simulink library "ddm"  (R2021b)
settings: Solver=VariableStepAuto  StartTime=0.0  StopTime=10.0  RelTol=1e-3
undefined symbols (not defined in the file or in its folder): ADDM_FrTMTqDev_X_Nm, ADDM_RrTMTqDev_X_Nm, ENUM_ADASACCSTA_ERROR, ENUM_ADASACCSTA_OFF, ENUM_ADASACCSTA_STANDBY, ENUM_ALLOWMOV_ALLOWREADY, ENUM_APS, ENUM_BRKSTA_ERROR, ENUM_BRKSTA_OFF, ENUM_BRKSTA_ON, ENUM_BRKSW_INVALID, ENUM_BRKSW_OFF, ENUM_BRKSW_ON, ENUM_CHGPREACTERRSTA_OBCPRE, ENUM_DCDCFAULTSTA_ANYFAULTLV1, ENUM_DCDCFAULTSTA_ANYFAULTLV2, ENUM_DRIVETRAIN_AWD, ENUM_DRIVETRAIN_FWD, ENUM_DRIVETRAIN_RWD, ENUM_EDUDRTSTA_NORMAL, ENUM_EPBSTA_APPLIED, ENUM_EPBSTA_RELEASED, ENUM_GEARACTUALPOSN_INVALID, ENUM_GEARACTUALPOSN_P, ENUM_HVBATTREADYPRE_READY, ENUM_MCUWARN_LV0, ENUM_MCUWARN_LV1, ENUM_MCUWARN_LV2, ENUM_MCUWARN_LV3, ENUM_MCUWARN_NOERROR, ENUM_OBCFAULTSTA_ANYFAULT, ENUM_PAS_R2F2, ENUM_PDFAULT_BATTPDFAIL, ENUM_PDFAULT_DCDCDISABLE, ENUM_PDFAULT_MCUDISABLE, ENUM_PDFAULT_MCUDISCHRG, ENUM_POWERSTA_OFF, ENUM_POWERSTA_ON, ENUM_POWERSTA_READY, ENUM_POWERSTA_STANDBY, ENUM_PRESSINDI_LOW, ENUM_PUFAULT_BATTUPFAIL, ENUM_PUFAULT_DCDCENABLEFAIL, ENUM_PUFAULT_PRECHRGCHKFAIL, ENUM_PUFAULT_SAFETYCHKFAIL, ENUM_PUSTATE_COMPLETED, ENUM_PWRSTASW_OFF, ENUM_PWRSTASW_OFFA, ENUM_PWRSTASW_OFFCHVCHRG, ENUM_PWRSTASW_OFFCLVCHRG, ENUM_PWRSTASW_ON, ENUM_PWRSTASW_ONHVCHRG, ENUM_PWRSTASW_READY, ENUM_PWRSTASW_STANDBY, ENUM_SHIFTCOMMAND_P, ENUM_SHIFTERERRSTA_PBUTTONFAILURE, ENUM_VEHMALFUNLV_2ND, ENUM_VEHMALFUNLV_3RD, ENUM_VEHMALFUNLV_4TH, ENUM_VEHMALFUNLV_NORMAL ... (+459)
libraries: hcu_lib x515, simulink x3
(part 9 of 25)

== system ddm/DDM/DDM/PMM/SW failure ==
  task_time_s : Inport
  VPMM_PwrStaSW_enum : Inport  Port=2
  VPMM_PowerSta_enum : Inport  Port=3
  DTC_clear_request : Inport  Port=4
  VINP_DrStSW : Inport  Port=5
  VINP_FLAJARSW : Inport  Port=6
  VINP_FRAJARSW : Inport  Port=7
  VINP_RLAJARSW : Inport  Port=8
  VINP_RRAJARSW : Inport  Port=9
  VINP_HoodSW : Inport  Port=10
  VINP_TailgaSW : Inport  Port=11
  Driver seat switch failure : Subsystem
  FL Door switch failure : Subsystem
  FR Door switch failure : Subsystem
  Hood switch failure : Subsystem
  RL Door switch failure : Subsystem
  RR Door switch failure : Subsystem
  Tailgate switch failure : Subsystem
  VDDM_DrStSWDTC_raw32 : Outport
  VDDM_FLDoorSWDTC_raw32 : Outport  Port=2
  VDDM_RLDoorSWDTC_raw32 : Outport  Port=3
  VDDM_FRDoorSWDTC_raw32 : Outport  Port=4
  VDDM_RRDoorSWDTC_raw32 : Outport  Port=5
  VDDM_HoodSWDTC_raw32 : Outport  Port=6
  VDDM_TailgaSWDTC_raw32 : Outport  Port=7
  VDDM_VCUFLDoorSta_flg : Outport  Port=8
  VDDM_VCUFRDoorSta_flg : Outport  Port=9
  VDDM_VCURLDoorSta_flg : Outport  Port=10
  VDDM_VCURRDoorSta_flg : Outport  Port=11
  VDDM_VCUHoodSWSta_flg : Outport  Port=12
  VDDM_VCUTailgateSWSta_flg : Outport  Port=13
  VDDM_DrStSWCFS_flg : Outport  Port=14
  VDDM_FLDoorSWCFS_flg : Outport  Port=15
  VDDM_RLDoorSWCFS_flg : Outport  Port=16
  VDDM_FRDoorSWCFS_flg : Outport  Port=17
  VDDM_RRDoorSWCFS_flg : Outport  Port=18
  VDDM_HoodSWCFS_flg : Outport  Port=19
  VDDM_TailgaSWCFS_flg : Outport  Port=20
  wires:
  Tailgate switch failure/2(VDDM_VCUTailgateSWSta_flg) -> VDDM_VCUTailgateSWSta_flg/1
  Tailgate switch failure/1(VDDM_TailgaSWDTC_raw32) -> VDDM_TailgaSWDTC_raw32/1
  [VINP_TailgaSW] -> Tailgate switch failure/4(VINP_TailgaSW)
  [DTC_clear_request] -> Tailgate switch failure/5(DTC_clear_request)
  [VPMM_PwrStaSW_enum] -> Tailgate switch failure/3(VPMM_PwrStaSW_enum)
  [VPMM_PowerSta_enum] -> Tailgate switch failure/2(VPMM_PowerSta_enum)
  [task_time_s] -> Tailgate switch failure/1(task_time_s)
  Hood switch failure/2(VDDM_VCUHoodSWSta_flg) -> VDDM_VCUHoodSWSta_flg/1
  Hood switch failure/1(VDDM_HoodSWDTC_raw32) -> VDDM_HoodSWDTC_raw32/1
  [DTC_clear_request] -> Hood switch failure/5(DTC_clear_request)
  [VINP_HoodSW] -> Hood switch failure/4(VINP_HoodSW)
  VINP_TailgaSW/1 -> [VINP_TailgaSW]
  VINP_HoodSW/1 -> [VINP_HoodSW]
  [VPMM_PwrStaSW_enum] -> Hood switch failure/3(VPMM_PwrStaSW_enum)
  [VPMM_PowerSta_enum] -> Hood switch failure/2(VPMM_PowerSta_enum)
  [task_time_s] -> Hood switch failure/1(task_time_s)
  RR Door switch failure/2(VDDM_VCURRDoorSta_flg) -> VDDM_VCURRDoorSta_flg/1
  RR Door switch failure/1(VDDM_RRDoorSWDTC_raw32) -> VDDM_RRDoorSWDTC_raw32/1
  [DTC_clear_request] -> RR Door switch failure/5(DTC_clear_request)
  [VINP_RRAJARSW] -> RR Door switch failure/4(VINP_RRAJARSW)
  [VPMM_PwrStaSW_enum] -> RR Door switch failure/3(VPMM_PwrStaSW_enum)
  [VPMM_PowerSta_enum] -> RR Door switch failure/2(VPMM_PowerSta_enum)
  [task_time_s] -> RR Door switch failure/1(task_time_s)
  RL Door switch failure/2(VDDM_VCURLDoorSta_flg) -> VDDM_VCURLDoorSta_flg/1
  RL Door switch failure/1(VDDM_RLDoorSWDTC_raw32) -> VDDM_RLDoorSWDTC_raw32/1
  [DTC_clear_request] -> RL Door switch failure/5(DTC_clear_request)
  [VINP_RLAJARSW] -> RL Door switch failure/4(VINP_RLAJARSW)
  [task_time_s] -> RL Door switch failure/1(task_time_s)
  [VPMM_PowerSta_enum] -> RL Door switch failure/2(VPMM_PowerSta_enum)
  [VPMM_PwrStaSW_enum] -> RL Door switch failure/3(VPMM_PwrStaSW_enum)
  FR Door switch failure/2(VDDM_VCUFRDoorSta_flg) -> VDDM_VCUFRDoorSta_flg/1
  FR Door switch failure/1(VDDM_FRDoorSWDTC_raw32) -> VDDM_FRDoorSWDTC_raw32/1
  [DTC_clear_request] -> FR Door switch failure/5(DTC_clear_request)
  [VINP_FRAJARSW] -> FR Door switch failure/4(VINP_FRAJARSW)
  [VPMM_PwrStaSW_enum] -> FR Door switch failure/3(VPMM_PwrStaSW_enum)
  [VPMM_PowerSta_enum] -> FR Door switch failure/2(VPMM_PowerSta_enum)
  [task_time_s] -> FR Door switch failure/1(task_time_s)
  FL Door switch failure/2(VDDM_VCUFLDoorSta_flg) -> VDDM_VCUFLDoorSta_flg/1
  FL Door switch failure/1(VDDM_FLDoorSWDTC_raw32) -> VDDM_FLDoorSWDTC_raw32/1
  [DTC_clear_request] -> FL Door switch failure/5(DTC_clear_request)
  [VINP_FLAJARSW] -> FL Door switch failure/4(VINP_FLAJARSW)
  [VPMM_PwrStaSW_enum] -> FL Door switch failure/3(VPMM_PwrStaSW_enum)
  [VPMM_PowerSta_enum] -> FL Door switch failure/2(VPMM_PowerSta_enum)
  [task_time_s] -> FL Door switch failure/1(task_time_s)
  VINP_RRAJARSW/1 -> [VINP_RRAJARSW]
  VINP_RLAJARSW/1 -> [VINP_RLAJARSW]
  VINP_FRAJARSW/1 -> [VINP_FRAJARSW]
  VINP_FLAJARSW/1 -> [VINP_FLAJARSW]
  Driver seat switch failure/2(VDDM_DrStSWCFS_flg) -> VDDM_DrStSWCFS_flg/1
  DTC_clear_request/1 -> [DTC_clear_request]
  VPMM_PowerSta_enum/1 -> [VPMM_PowerSta_enum]
  VPMM_PwrStaSW_enum/1 -> [VPMM_PwrStaSW_enum]
  task_time_s/1 -> [task_time_s]
  VINP_DrStSW/1 -> [VINP_DrStSW]
  [task_time_s] -> Driver seat switch failure/1(task_time_s)
  [VINP_DrStSW] -> Driver seat switch failure/4(VINP_DrStSW)
  [DTC_clear_request] -> Driver seat switch failure/5(DTC_clear_request)
  [VPMM_PwrStaSW_enum] -> Driver seat switch failure/3(VPMM_PwrStaSW_enum)
  [VPMM_PowerSta_enum] -> Driver seat switch failure/2(VPMM_PowerSta_enum)
  Driver seat switch failure/1(VDDM_DrStSWDTC_raw32) -> VDDM_DrStSWDTC_raw32/1
  FL Door switch failure/3(VDDM_FLDoorSWCFS_flg) -> VDDM_FLDoorSWCFS_flg/1
  RL Door switch failure/3(VDDM_RLDoorSWCFS_flg) -> VDDM_RLDoorSWCFS_flg/1
  FR Door switch failure/3(VDDM_FRDoorSWCFS_flg) -> VDDM_FRDoorSWCFS_flg/1
  RR Door switch failure/3(VDDM_RRDoorSWCFS_flg) -> VDDM_RRDoorSWCFS_flg/1
  Hood switch failure/3(VDDM_HoodSWCFS_flg) -> VDDM_HoodSWCFS_flg/1
  Tailgate switch failure/3(VDDM_TailgaSWCFS_flg) -> VDDM_TailgaSWCFS_flg/1

== system ddm/DDM/DDM/PMM/System conditions of ON to READY not satisfied ==
  note: Release Condition After Decision
  note: Test Detection Criteria
  note: Diagnostics and Fault Handling
  note: Test Pass Criteria
  task_time_s : Inport
  VPMM_PowerSta_enum : Inport  Port=2
  VPMM_PwrStaSW_enum : Inport  Port=3
  DTC_clear_request : Inport  Port=4
  VPMM_MCUReady_flg : Inport  Port=5
  VINP_AllowMovThd_OTA_enum : Inport  Port=6
  VDDM_KeyAuthCFS_flg : Inport  Port=7
  VDDM_FLDoorSWCFS_flg : Inport  Port=8
  VDDM_RLDoorSWCFS_flg : Inport  Port=9
  VDDM_FRDoorSWCFS_flg : Inport  Port=10
  VDDM_RRDoorSWCFS_flg : Inport  Port=11
  VDDM_HoodSWCFS_flg : Inport  Port=12
  VDDM_TailgaSWCFS_flg : Inport  Port=13
  Constant{1..2,9,12,22} (5 alike) : Constant  Value=FALSE
  Constant10 : Constant  Value=ENUM_POWERSTA_STANDBY
  Constant13 : Constant  Value=KDDM_ONtoRdyPassTO_s
  Constant14 : Constant  Value=KDDM_ONtoRdyPassTO_s
  Constant17 : Constant  Value=KDDM_ONtoRdyDetTO_s
  Constant18 : Constant  Value=KDDM_ONtoRdyDTC_cnt
  Constant28 : Constant  Value=ENUM_PWRSTASW_ON
  Constant29 : Constant  Value=ENUM_PWRSTASW_ON
  Constant3 : Constant  Value=TRUE
  Constant30 : Constant  Value=KDDM_ONtoRdyDiagnosisOffSW_flg
  Constant31 : Constant  Value=ENUM_POWERSTA_OFF
  Constant32 : Constant  Value=ENUM_ALLOWMOV_ALLOWREADY
  Constant34 : Constant  Value=ZERO_INT
  Constant35 : Constant  Value=KDDM_ONtoRdyDTC_cnt
  Constant4 : Constant  Value=TRUE
  Constant5 : Constant  Value=ENUM_ALLOWMOV_ALLOWREADY
  DTC_Couter1 : hcu_lib/Basic_Blocks/DTC_Couter
  DTC_Info : hcu_lib/Basic_Blocks/DTC_Info
  Equal1 : RelationalOperator  Operator=~=  OutDataTypeStr=boolean  RndMeth=Simplest
  Equal{8,10,12,14} (4 alike) : RelationalOperator  Operator===  OutDataTypeStr=boolean  RndMeth=Simplest
  Equal11 : RelationalOperator  Operator=~=  OutDataTypeStr=boolean  RndMeth=Simplest
  Equal13 : RelationalOperator  OutDataTypeStr=boolean  RndMeth=Simplest
  Logical Operator1 : Logic  Operator=NOT  AllPortsSameDT=off  OutDataTypeStr=boolean
  Logical Operator14 : Logic  Operator=NOT  AllPortsSameDT=off  OutDataTypeStr=boolean
  Logical Operator16 : Logic  Operator=OR  Inputs=4  AllPortsSameDT=off  OutDataTypeStr=boolean
  Logical Operator17 : Logic  AllPortsSameDT=off  OutDataTypeStr=boolean
  Logical Operator2 : Logic  Operator=OR  Inputs=9  AllPortsSameDT=off  OutDataTypeStr=boolean
  Logical Operator20 : Logic  Operator=OR  Inputs=9  AllPortsSameDT=off  OutDataTypeStr=boolean
  Logical Operator21 : Logic  Operator=NOT  AllPortsSameDT=off  OutDataTypeStr=boolean
  Relational Operator1 : RelationalOperator  Operator=>  OutDataTypeStr=boolean  RndMeth=Simplest
  Switch{1..4,9} (5 alike) : Switch  Criteria=u2 ~= 0
  Terminator : Terminator
  Test Detection Criteria1 : hcu_lib/Basic_Blocks/Test Detection Criteria
  Timer2 : hcu_lib/Basic_Blocks/Timer
  Unit Delay1 : UnitDelay  SampleTime=-1  HasFrameUpgradeWarning=on
  VDDM_ONtoRdyDTC_raw32 : Outport
  VDDM_ONtoRdyCFS_flg : Outport  Port=2
  VDDM_EDriveSysErrONtoRdy_flg : Outport  Port=3
  VDDM_SysAllowReadySta_flg : Outport  Port=4
  wires:
  [VDDM_RRDoorSWCFS_flg] -> Logical Operator2/7
  Logical Operator2/1 -> Switch3/1
  [VDDM_FRDoorSWCFS_flg] -> Logical Operator2/6
  [VDDM_RLDoorSWCFS_flg] -> Logical Operator2/5
  [VDDM_FLDoorSWCFS_flg] -> Logical Operator2/4
  [VPMM_MCUReady_flg] -> Logical Operator1/1
  [VDDM_TailgaSWCFS_flg] -> Logical Operator2/9
  [VDDM_HoodSWCFS_flg] -> Logical Operator2/8
  [VDDM_KeyAuthCFS_flg] -> Logical Operator2/3
  Equal1/1 -> Logical Operator2/2
  Constant5/1 -> Equal1/2
  [VINP_AllowMovThd_OTA_enum] -> Equal1/1
  Logical Operator1/1 -> Logical Operator2/1
  [VDDM_TailgaSWCFS_flg] -> Logical Operator20/9
  [VDDM_HoodSWCFS_flg] -> Logical Operator20/8
  [VDDM_RRDoorSWCFS_flg] -> Logical Operator20/7
  [VDDM_FRDoorSWCFS_flg] -> Logical Operator20/6
  [VDDM_RLDoorSWCFS_flg] -> Logical Operator20/5
  [VDDM_FLDoorSWCFS_flg] -> Logical Operator20/4
  VDDM_TailgaSWCFS_flg/1 -> [VDDM_TailgaSWCFS_flg]
  VDDM_HoodSWCFS_flg/1 -> [VDDM_HoodSWCFS_flg]
  VDDM_RRDoorSWCFS_flg/1 -> [VDDM_RRDoorSWCFS_flg]
  VDDM_FRDoorSWCFS_flg/1 -> [VDDM_FRDoorSWCFS_flg]
  VDDM_RLDoorSWCFS_flg/1 -> [VDDM_RLDoorSWCFS_flg]
  VDDM_FLDoorSWCFS_flg/1 -> [VDDM_FLDoorSWCFS_flg]
  Switch4/1 -> VDDM_SysAllowReadySta_flg/1  "VDDM_SysAllowReadySta_flg"
  Constant1/1 -> Switch4/3
  Constant4/1 -> Switch4/1
  [VDDM_ONtoRdyCFS_flg] -> Switch4/2
  Switch2/1 -> VDDM_EDriveSysErrONtoRdy_flg/1  "VDDM_EDriveSysErrONtoRdy_flg"
  Constant3/1 -> Switch2/1
  Constant2/1 -> Switch2/3
  [VDDM_ONtoRdyCFS_flg] -> Switch2/2
  [VDDM_ONtoRdyCFS_flg] -> VDDM_ONtoRdyCFS_flg/1
  [VPMM_PwrStaSW_enum] -> Equal12/1
  Constant29/1 -> Equal12/2
  Constant9/1 -> Switch3/3
  Equal12/1 -> Switch3/2
  Constant32/1 -> Equal11/2
  [VDDM_KeyAuthCFS_flg] -> Logical Operator20/3
  Equal11/1 -> Logical Operator20/2
  Logical Operator14/1 -> Logical Operator20/1
  [VPMM_MCUReady_flg] -> Logical Operator14/1
  [VINP_AllowMovThd_OTA_enum] -> Equal11/1
  Logical Operator16/1 -> [VDDM_ONtoRdyCFSRls_flg]  "VDDM_ONtoRdyCFSRls_flg"
  [VDDM_ONtoRdyCFSRls_flg] -> DTC_Couter1/2
  [VDDM_ONtoRdyDet_flg] -> DTC_Couter1/1
  DTC_Couter1/1 -> [VDDM_ONtoRdyCFS_flg]  "VDDM_ONtoRdyCFS_flg"
  Constant14/1 -> Equal13/2
  [VDDM_ONtoRdyCFSRls_flg] -> Switch9/2
  Unit Delay1/1 -> Equal14/1
  Relational Operator1/1 -> Terminator/1  "VDDM_ONtoRdyDFS_flg"
  Constant34/1 -> Relational Operator1/2
  [VPMM_PowerSta_enum] -> Unit Delay1/1
  Equal14/1 -> Logical Operator17/1
  Switch3/1 -> Logical Operator21/1, Timer2/2
  Constant30/1 -> Logical Operator16/4
  Switch9/1 -> Test Detection Criteria1/1
  [task_time_s] -> Test Detection Criteria1/2
  [task_time_s] -> Timer2/3
  Switch1/1 -> Switch9/3
  Logical Operator21/1 -> Timer2/1
  Logical Operator17/1 -> Logical Operator16/1
  Constant12/1 -> Switch1/3
  Equal10/1 -> Logical Operator17/2
  Constant31/1 -> Equal14/2
  [DTC_clear_request] -> Logical Operator16/2
  DTC_Couter1/2 -> Relational Operator1/1  "VDDM_ONtoRdyDTC_cnt"
  Logical Operator20/1 -> Switch1/1
  [VPMM_PowerSta_enum] -> Equal10/1
  Constant22/1 -> Switch9/1
  Timer2/1 -> Equal13/1
  Constant10/1 -> Equal10/2
  Test Detection Criteria1/1 -> [VDDM_ONtoRdyDet_flg]  "VDDM_ONtoRdyDet_flg"
  Equal8/1 -> Switch1/2
  Constant13/1 -> Timer2/4
  Constant18/1 -> Test Detection Criteria1/3
  Constant35/1 -> DTC_Couter1/3
  [VPMM_PwrStaSW_enum] -> Equal8/1
  Equal13/1 -> [VDDM_ONtoRdyPass_flg]  "VDDM_ONtoRdyPass_flg"
  Constant28/1 -> Equal8/2
  Constant17/1 -> Test Detection Criteria1/4
  [VDDM_ONtoRdyPass_flg] -> Logical Operator16/3
  DTC_clear_request/1 -> [DTC_clear_request]
  task_time_s/1 -> [task_time_s]
  VPMM_PwrStaSW_enum/1 -> [VPMM_PwrStaSW_enum]
  VPMM_PowerSta_enum/1 -> [VPMM_PowerSta_enum]
  VPMM_MCUReady_flg/1 -> [VPMM_MCUReady_flg]
  VINP_AllowMovThd_OTA_enum/1 -> [VINP_AllowMovThd_OTA_enum]
  DTC_Info/1 -> VDDM_ONtoRdyDTC_raw32/1  "VDDM_ONtoRdyDTC_raw32"
  [VDDM_ONtoRdyPass_flg] -> DTC_Info/2
  [VDDM_ONtoRdyCFS_flg] -> DTC_Info/3
  VDDM_KeyAuthCFS_flg/1 -> [VDDM_KeyAuthCFS_flg]
  [VDDM_ONtoRdyDet_flg] -> DTC_Info/1
  [DTC_clear_request] -> DTC_Info/4

== system ddm/DDM/DDM/PMM/power up and power down ==
  note: Power up fail check
  note: Power down fail check
  note: OBC ready for precharge fail check
  task_time_s : Inport
  VPMM_PwrStaSW_enum : Inport  Port=2
  VPMM_PowerSta_enum : Inport  Port=3
  VPMM_PowerUpFault_enum : Inport  Port=4
  VPMM_PowerDownFault_enum : Inport  Port=5
  DTC_clear_request : Inport  Port=6
  VINP_HVBattReady4Pre_enum : Inport  Port=7
  VPMM_MCUReady4Pre_flg : Inport  Port=8
  VINP_DCDCReady4Pre_flg : Inport  Port=9
  VINP_HVBContactorSta_flg : Inport  Port=10
  VINP_BMSREADY_flg : Inport  Port=11
  VINP_DCDCEnabled_flg : Inport  Port=12
  VPMM_SafetyChkHLv_flg : Inport  Port=13
  VPMM_SafetyChkMLv_flg : Inport  Port=14
  VPMM_HVChrgPreActionErrSta_enum : Inport  Port=15
  VPMM_PowerUpState_enum : Inport  Port=16
  VPMM_MCUDCBusMaxVolt_V : Inport  Port=17
  BMS HV relay closed fail : Subsystem
  BMS HV relay opened fail : Subsystem
  BMS ready fail : Subsystem
  DCDC disable fail : Subsystem
  DCDC enable fail : Subsystem
  DCDC ready for precharge fail : Subsystem
  HVB ready for precharge fail : Subsystem
  High level system safety check fail : Subsystem
  MCU active discharge fail : Subsystem
  MCU disable fail : Subsystem
  MCU ready for precharge fail : Subsystem
  Mid level system safety check fail : Subsystem
  OBC ready for precharge fail : Subsystem
  VDDM_HVB4PreDTC_raw32 : Outport
  VDDM_MCU4PreDTC_raw32 : Outport  Port=2
  VDDM_DCDC4PreDTC_raw32 : Outport  Port=3
  VDDM_HVRlyCloDTC_raw32 : Outport  Port=4
  VDDM_BMSRdyDTC_raw32 : Outport  Port=5
  VDDM_DCDCEnaDTC_raw32 : Outport  Port=6
  VDDM_HiLvSaChkDTC_raw32 : Outport  Port=7
  VDDM_MidLvSaChkDTC_raw32 : Outport  Port=8
  VDDM_MCUDisDTC_raw32 : Outport  Port=9
  VDDM_DCDCDisDTC_raw32 : Outport  Port=10
  VDDM_HVRlyOpDTC_raw32 : Outport  Port=11
  VDDM_MCUActDTC_raw32 : Outport  Port=12
  VDDM_OBC4PreDTC_raw32 : Outport  Port=13
  VDDM_HVRlyOpFail_flg : Outport  Port=14
  VDDM_MCUActDisFail_flg : Outport  Port=15
  VDDM_HVB4PreCFS_flg : Outport  Port=16
  VDDM_MCU4PreCFS_flg : Outport  Port=17
  VDDM_DCDC4PreCFS_flg : Outport  Port=18
  VDDM_HVRlyCloCFS_flg : Outport  Port=19
  VDDM_BMSRdyCFS_flg : Outport  Port=20
  VDDM_DCDCEnaCFS_flg : Outport  Port=21
  VDDM_HiLvSaChkCFS_flg : Outport  Port=22
  VDDM_MidLvSaChkCFS_flg : Outport  Port=23
  VDDM_MCUDisCFS_flg : Outport  Port=24
  VDDM_DCDCDisCFS_flg : Outport  Port=25
  VDDM_HVRlyOpCFS_flg : Outport  Port=26
  VDDM_MCUActCFS_flg : Outport  Port=27
  VDDM_OBC4PreCFS_flg : Outport  Port=28
  wires:
  [VPMM_PowerUpState_enum] -> Mid level system safety check fail/7(VPMM_PowerUpState_enum)
  [VPMM_PowerUpState_enum] -> BMS HV relay closed fail/7(VPMM_PowerUpState_enum)
  [VPMM_PowerUpState_enum] -> High level system safety check fail/7(VPMM_PowerUpState_enum)
  [VPMM_PowerUpState_enum] -> DCDC ready for precharge fail/7(VPMM_PowerUpState_enum)
  [VPMM_PowerUpState_enum] -> DCDC enable fail/7(VPMM_PowerUpState_enum)
  [VPMM_PowerUpState_enum] -> MCU ready for precharge fail/7(VPMM_PowerUpState_enum)
  [VPMM_PowerUpState_enum] -> BMS ready fail/7(VPMM_PowerUpState_enum)
  [VPMM_PowerUpState_enum] -> HVB ready for precharge fail/7(VPMM_PowerUpState_enum)
  VPMM_PowerUpState_enum/1 -> [VPMM_PowerUpState_enum]
  BMS HV relay closed fail/1(VDDM_HVRlyCloDTC_raw32) -> VDDM_HVRlyCloDTC_raw32/1
  DCDC ready for precharge fail/1(VDDM_DCDC4PreDTC_raw32) -> VDDM_DCDC4PreDTC_raw32/1
  MCU ready for precharge fail/1(VDDM_MCU4PreDTC_raw32) -> VDDM_MCU4PreDTC_raw32/1
  HVB ready for precharge fail/1(VDDM_HVB4PreDTC_raw32) -> VDDM_HVB4PreDTC_raw32/1
  MCU active discharge fail/2(VDDM_MCUActDisFail_flg) -> VDDM_MCUActDisFail_flg/1
  BMS HV relay opened fail/2(VDDM_HVRlyOpFail_flg) -> VDDM_HVRlyOpFail_flg/1
  [VINP_HVBContactorSta_flg] -> BMS HV relay closed fail/4(VINP_HVBContactorSta_flg)
  VINP_HVBContactorSta_flg/1 -> [VINP_HVBContactorSta_flg]
  [VPMM_PowerDownFault_enum] -> MCU active discharge fail/4(VPMM_PowerDownFault_enum)
  [VPMM_PowerDownFault_enum] -> BMS HV relay opened fail/4(VPMM_PowerDownFault_enum)
  [VPMM_PowerDownFault_enum] -> DCDC disable fail/4(VPMM_PowerDownFault_enum)
  [VINP_DCDCEnabled_flg] -> DCDC enable fail/4(VINP_DCDCEnabled_flg)
  VINP_DCDCEnabled_flg/1 -> [VINP_DCDCEnabled_flg]
  [VPMM_PowerDownFault_enum] -> MCU disable fail/4(VPMM_PowerDownFault_enum)
  VPMM_PowerDownFault_enum/1 -> [VPMM_PowerDownFault_enum]
  [VPMM_PowerUpFault_enum] -> Mid level system safety check fail/5(VPMM_PowerUpFault_enum)
  VPMM_SafetyChkMLv_flg/1 -> Mid level system safety check fail/4(VDDM_MidLvSaChkChk_flg)
  High level system safety check fail/1(VDDM_HiLvSaChkDTC_raw32) -> VDDM_HiLvSaChkDTC_raw32/1
  VPMM_SafetyChkHLv_flg/1 -> High level system safety check fail/4(VPMM_SafetyChkHLv_flg)
  [VPMM_PowerSta_enum] -> High level system safety check fail/3(VPMM_PwrStaSW_enum)
  [DTC_clear_request] -> High level system safety check fail/6(DTC_clear_request)
  [VPMM_PowerUpFault_enum] -> High level system safety check fail/5(VPMM_PowerUpFault_enum)
  [VPMM_PwrStaSW_enum] -> High level system safety check fail/2(VPMM_PowerSta_enum)
  [task_time_s] -> High level system safety check fail/1(task_time_s)
  DCDC enable fail/1(VDDM_DCDCEnaDTC_raw32) -> VDDM_DCDCEnaDTC_raw32/1
  [VPMM_PowerSta_enum] -> DCDC enable fail/3(VPMM_PwrStaSW_enum)
  [VPMM_PwrStaSW_enum] -> DCDC enable fail/2(VPMM_PowerSta_enum)
  [DTC_clear_request] -> DCDC enable fail/6(DTC_clear_request)
  [VPMM_PowerUpFault_enum] -> DCDC enable fail/5(VPMM_PowerUpFault_enum)
  [task_time_s] -> DCDC enable fail/1(task_time_s)
  BMS ready fail/1(VDDM_BMSRdyDTC_raw32) -> VDDM_BMSRdyDTC_raw32/1
  VINP_BMSREADY_flg/1 -> BMS ready fail/4(VINP_BMSREADY_flg)
  [VPMM_PowerSta_enum] -> BMS ready fail/3(VPMM_PwrStaSW_enum)
  [VPMM_PwrStaSW_enum] -> BMS ready fail/2(VPMM_PowerSta_enum)
  [DTC_clear_request] -> BMS ready fail/6(DTC_clear_request)
  [VPMM_PowerUpFault_enum] -> BMS ready fail/5(VPMM_PowerUpFault_enum)
  [task_time_s] -> BMS ready fail/1(task_time_s)
  [VPMM_PowerUpFault_enum] -> BMS HV relay closed fail/5(VPMM_PowerUpFault_enum)
  [VPMM_PowerUpFault_enum] -> DCDC ready for precharge fail/5(VPMM_PowerUpFault_enum)
  [VPMM_PowerUpFault_enum] -> MCU ready for precharge fail/5(VPMM_PowerUpFault_enum)
  [DTC_clear_request] -> MCU ready for precharge fail/6(DTC_clear_request)
  VPMM_MCUReady4Pre_flg/1 -> MCU ready for precharge fail/4(VPMM_MCUReady4Pre_flg)
  [VPMM_PowerUpFault_enum] -> HVB ready for precharge fail/5(VPMM_PowerUpFault_enum)
  VPMM_HVChrgPreActionErrSta_enum/1 -> OBC ready for precharge fail/4(VPMM_HVChrgPreActionErrSta_enum)
  VINP_DCDCReady4Pre_flg/1 -> DCDC ready for precharge fail/4(VINP_DCDCReady4Pre_flg)
  VINP_HVBattReady4Pre_enum/1 -> HVB ready for precharge fail/4(VINP_HVBattReady4Pre_enum)
  MCU active discharge fail/1(VDDM_MCUActDTC_raw32) -> VDDM_MCUActDTC_raw32/1
  MCU disable fail/1(VDDM_MCUDisDTC_raw32) -> VDDM_MCUDisDTC_raw32/1
  Mid level system safety check fail/1(VDDM_MidLvSaChkDTC_raw32) -> VDDM_MidLvSaChkDTC_raw32/1
  BMS HV relay opened fail/1(VDDM_HVRlyOpDTC_raw32) -> VDDM_HVRlyOpDTC_raw32/1
  OBC ready for precharge fail/1(VDDM_OBC4PreDTC_raw32) -> VDDM_OBC4PreDTC_raw32/1
  DCDC disable fail/1(VDDM_DCDCDisDTC_raw32) -> VDDM_DCDCDisDTC_raw32/1
  [VPMM_PowerSta_enum] -> OBC ready for precharge fail/3(VPMM_PwrStaSW_enum)
  [DTC_clear_request] -> OBC ready for precharge fail/5(DTC_clear_request)
  [VPMM_PwrStaSW_enum] -> OBC ready for precharge fail/2(VPMM_PowerSta_enum)
  [task_time_s] -> OBC ready for precharge fail/1(task_time_s)
  [task_time_s] -> MCU active discharge fail/1(task_time_s)
  [VPMM_PwrStaSW_enum] -> MCU active discharge fail/3(VPMM_PwrStaSW_enum)
  [DTC_clear_request] -> MCU active discharge fail/5(DTC_clear_request)
  [VPMM_PowerSta_enum] -> MCU active discharge fail/2(VPMM_PowerSta_enum)
  [VPMM_PowerSta_enum] -> BMS HV relay opened fail/2(VPMM_PowerSta_enum)
  [DTC_clear_request] -> BMS HV relay opened fail/5(DTC_clear_request)
  [VPMM_PwrStaSW_enum] -> BMS HV relay opened fail/3(VPMM_PwrStaSW_enum)
  [task_time_s] -> BMS HV relay opened fail/1(task_time_s)
  [task_time_s] -> DCDC disable fail/1(task_time_s)
  [VPMM_PwrStaSW_enum] -> DCDC disable fail/2(VPMM_PowerSta_enum)
  [DTC_clear_request] -> DCDC disable fail/5(DTC_clear_request)
  [VPMM_PowerSta_enum] -> DCDC disable fail/3(VPMM_PwrStaSW_enum)
  [VPMM_PowerSta_enum] -> MCU disable fail/3(VPMM_PwrStaSW_enum)
  [DTC_clear_request] -> MCU disable fail/5(DTC_clear_request)
  [VPMM_PwrStaSW_enum] -> MCU disable fail/2(VPMM_PowerSta_enum)
  [task_time_s] -> MCU disable fail/1(task_time_s)
  [task_time_s] -> Mid level system safety check fail/1(task_time_s)
  [VPMM_PwrStaSW_enum] -> Mid level system safety check fail/2(VPMM_PowerSta_enum)
  [DTC_clear_request] -> Mid level system safety check fail/6(DTC_clear_request)
  [VPMM_PowerSta_enum] -> Mid level system safety check fail/3(VPMM_PwrStaSW_enum)
  DTC_clear_request/1 -> [DTC_clear_request]
  VPMM_PowerSta_enum/1 -> [VPMM_PowerSta_enum]
  task_time_s/1 -> [task_time_s]
  VPMM_PwrStaSW_enum/1 -> [VPMM_PwrStaSW_enum]
  VPMM_PowerUpFault_enum/1 -> [VPMM_PowerUpFault_enum]
  [task_time_s] -> MCU ready for precharge fail/1(task_time_s)
  [VPMM_PwrStaSW_enum] -> HVB ready for precharge fail/2(VPMM_PowerSta_enum)
  [VPMM_PwrStaSW_enum] -> BMS HV relay closed fail/2(VPMM_PowerSta_enum)
  [VPMM_PowerSta_enum] -> BMS HV relay closed fail/3(VPMM_PwrStaSW_enum)
  [task_time_s] -> BMS HV relay closed fail/1(task_time_s)
  [VPMM_PowerSta_enum] -> MCU ready for precharge fail/3(VPMM_PwrStaSW_enum)
  [VPMM_PwrStaSW_enum] -> DCDC ready for precharge fail/2(VPMM_PowerSta_enum)
  [task_time_s] -> DCDC ready for precharge fail/1(task_time_s)
  [DTC_clear_request] -> DCDC ready for precharge fail/6(VINP_ReqClrDTC_flg)
  [task_time_s] -> HVB ready for precharge fail/1(task_time_s)
  [DTC_clear_request] -> HVB ready for precharge fail/6(DTC_clear_request)
  [VPMM_PowerSta_enum] -> HVB ready for precharge fail/3(VPMM_PwrStaSW_enum)
  [VPMM_PowerSta_enum] -> DCDC ready for precharge fail/3(VPMM_PwrStaSW_enum)
  [VPMM_PwrStaSW_enum] -> MCU ready for precharge fail/2(VPMM_PowerSta_enum)
  [DTC_clear_request] -> BMS HV relay closed fail/6(DTC_clear_request)
  [VPMM_MCUDCBusMaxVolt_V] -> MCU active discharge fail/6(VPMM_MCUDCBusMaxVolt_V)
  HVB ready for precharge fail/2(VDDM_HVB4PreCFS_flg) -> [VDDM_HVB4PreCFS_flg]
  MCU ready for precharge fail/2(VDDM_MCU4PreCFS_flg) -> [VDDM_MCU4PreCFS_flg]
  DCDC ready for precharge fail/2(VDDM_DCDC4PreCFS_flg) -> [VDDM_DCDC4PreCFS_flg]
  BMS HV relay closed fail/2(VDDM_HVRlyCloCFS_flg) -> [VDDM_HVRlyCloCFS_flg]
  BMS ready fail/2(VDDM_BMSRdyCFS_flg) -> [VDDM_BMSRdyCFS_flg]
  DCDC enable fail/2(VDDM_DCDCEnaCFS_flg) -> [VDDM_DCDCEnaCFS_flg]
  High level system safety check fail/2(VDDM_HiLvSaChkCFS_flg) -> [VDDM_HiLvSaChkCFS_flg]
  Mid level system safety check fail/2(VDDM_MidLvSaChkCFS_flg) -> [VDDM_MidLvSaChkCFS_flg]
  MCU disable fail/2(VDDM_MCUDisCFS_flg) -> [VDDM_MCUDisCFS_flg]
  DCDC disable fail/2(VDDM_DCDCDisCFS_flg) -> [VDDM_DCDCDisCFS_flg]
  BMS HV relay opened fail/3(VDDM_HVRlyOpCFS_flg) -> [VDDM_HVRlyOpCFS_flg]
  MCU active discharge fail/3(VDDM_MCUActCFS_flg) -> [VDDM_MCUActCFS_flg]
  OBC ready for precharge fail/2(VDDM_OBC4PreCFS_flg) -> [VDDM_OBC4PreCFS_flg]
  [VDDM_HVB4PreCFS_flg] -> VDDM_HVB4PreCFS_flg/1
  [VDDM_MCU4PreCFS_flg] -> VDDM_MCU4PreCFS_flg/1
  [VDDM_DCDC4PreCFS_flg] -> VDDM_DCDC4PreCFS_flg/1
  [VDDM_HVRlyCloCFS_flg] -> VDDM_HVRlyCloCFS_flg/1
  [VDDM_BMSRdyCFS_flg] -> VDDM_BMSRdyCFS_flg/1
  [VDDM_DCDCEnaCFS_flg] -> VDDM_DCDCEnaCFS_flg/1
  [VDDM_HiLvSaChkCFS_flg] -> VDDM_HiLvSaChkCFS_flg/1
  [VDDM_MidLvSaChkCFS_flg] -> VDDM_MidLvSaChkCFS_flg/1
  [VDDM_MCUDisCFS_flg] -> VDDM_MCUDisCFS_flg/1
  [VDDM_DCDCDisCFS_flg] -> VDDM_DCDCDisCFS_flg/1
  [VDDM_HVRlyOpCFS_flg] -> VDDM_HVRlyOpCFS_flg/1
  [VDDM_MCUActCFS_flg] -> VDDM_MCUActCFS_flg/1
  [VDDM_OBC4PreCFS_flg] -> VDDM_OBC4PreCFS_flg/1
  VPMM_MCUDCBusMaxVolt_V/1 -> [VPMM_MCUDCBusMaxVolt_V]

== system ddm/DDM/DDM/TPM/LFBatwarn ==
  note: Test Detection Criteria
  note: Test Pass Criteria
  note: Release Condition After Decision
  note: Diagnostics and Fault Handling
  task_time_s : Inport
  VPMM_PowerSta_enum : Inport  Port=2
  DTC_clear_request : Inport  Port=3
  VTPM_LFBatwarn_flg : Inport  Port=4
  Constant : Constant  Value=KDDM_LFBatwarnDTC_cnt
  Constant1 : Constant  Value=KDDM_LFBatwarnDTC_cnt
  Constant10 : Constant  Value=ENUM_POWERSTA_OFF
  Constant11 : Constant  Value=KDDM_LFBatwarnPassSW_flg
  Constant12 : Constant  Value=FALSE
  Constant13 : Constant  Value=KDDM_LFBatwarnCFSSW_flg
  Constant14 : Constant  Value=KDDM_LFBatwarnDFSSW_flg
  Constant15 : Constant  Value=KDDM_LFBatwarnPassTO_s
  Constant2 : Constant  Value=ENUM_POWERSTA_READY
  Constant24 : Constant  Value=TRUE
  Constant25 : Constant  Value=FALSE
  Constant3 : Constant  Value=ENUM_POWERSTA_ON
  Constant4 : Constant  Value=FALSE
  Constant46 : Constant  Value=KDDM_LFBatwarnDetSW_flg
  Constant5 : Constant  Value=ENUM_POWERSTA_READY
  Constant6 : Constant  Value=KDDM_LFBatwarnDetTO_s
  Constant7 : Constant  Value=ENUM_POWERSTA_ON
  Constant8 : Constant  Value=TRUE
  Constant9 : Constant  Value=KDDM_LFBatwarnPassTO_s
  DTC_Couter : hcu_lib/Basic_Blocks/DTC_Couter
  DTC_Info : hcu_lib/Basic_Blocks/DTC_Info
  Data Type Conversion1 : DataTypeConversion  OutDataTypeStr=uint8
  Equal{1..5} (5 alike) : RelationalOperator  Operator===  OutDataTypeStr=boolean  RndMeth=Simplest
  Equal6 : RelationalOperator  OutDataTypeStr=boolean  RndMeth=Simplest
  Logical Operator{1,4..5,7..8} (5 alike) : Logic  Operator=OR  AllPortsSameDT=off  OutDataTypeStr=boolean
  Logical Operator12 : Logic  AllPortsSameDT=off  OutDataTypeStr=boolean
  Logical Operator15 : Logic  AllPortsSameDT=off  OutDataTypeStr=boolean
  Logical Operator18 : Logic  AllPortsSameDT=off  OutDataTypeStr=boolean
  Logical Operator19 : Logic  Inputs=3  AllPortsSameDT=off  OutDataTypeStr=boolean
  Logical Operator2 : Logic  Operator=NOT  AllPortsSameDT=off  OutDataTypeStr=boolean
  Logical Operator3 : Logic  Operator=OR  Inputs=3  AllPortsSameDT=off  OutDataTypeStr=boolean
  Logical Operator6 : Logic  Operator=NOT  AllPortsSameDT=off  OutDataTypeStr=boolean
  Relay : Relay  OnSwitchValue=ONE_INT  OffSwitchValue=ZERO_INT
  SR_Latch1 : Subsystem  mask(SR_Latch){}
      mask help: SR latch function.
  SR_Latch3 : hcu_lib/Basic_Blocks/SR_Latch
  SR_Latch4 : hcu_lib/Basic_Blocks/SR_Latch
  Switch{2..4,6} (4 alike) : Switch  Criteria=u2 ~= 0
  Test Detection Criteria : hcu_lib/Basic_Blocks/Test Detection Criteria
  Timer1 : hcu_lib/Basic_Blocks/Timer
  VDDM_LFBatwarnDTC_raw32 : Outport
  wires:
  task_time_s/1 -> [task_time_s]
  VPMM_PowerSta_enum/1 -> [VPMM_PowerSta_enum]
  Logical Operator8/1 -> Switch2/2
  Constant25/1 -> Switch2/3
  Switch2/1 -> [VDDM_LFBatwarnCFSRls_flg]
  [DTC_clear_request] -> Logical Operator8/2
  Constant24/1 -> Switch2/1
  Constant10/1 -> Equal4/2
  Equal4/1 -> Logical Operator8/1
  [VDDM_LFBatwarnDTC_cnt] -> Relay/1
  [VDDM_LFBatwarnCFS_flg] -> Logical Operator7/1
  Logical Operator3/1 -> Logical Operator15/1
  [VDDM_LFBatwarnDet_flg] -> Logical Operator19/1
  Relay/1 -> SR_Latch3/1
  DTC_Couter/2 -> Data Type Conversion1/1
  Logical Operator15/1 -> DTC_Couter/2
  Constant11/1 -> Logical Operator15/2
  Logical Operator19/1 -> DTC_Couter/1
  Constant46/1 -> Logical Operator19/2
  Data Type Conversion1/1 -> [VDDM_LFBatwarnDTC_cnt]  "VDDM_LFBatwarnDTC_cnt"
  DTC_Couter/1 -> SR_Latch4/1
  [VDDM_LFBatwarnPass_flg] -> Logical Operator3/2
  [VDDM_LFBatwarnCFSRls_flg] -> Logical Operator5/1
  SR_Latch4/1 -> Logical Operator18/1
  Logical Operator12/1 -> [VDDM_LFBatwarnDFS_flg]
  Constant13/1 -> Logical Operator18/2
  SR_Latch3/1 -> Logical Operator12/2
  Constant14/1 -> Logical Operator12/1
  Logical Operator18/1 -> [VDDM_LFBatwarnCFS_flg]
  [VDDM_LFBatwarnCFSRls_flg] -> Logical Operator3/3
  DTC_clear_request/1 -> [DTC_clear_request]
  [VPMM_PowerSta_enum] -> Equal4/1
  [VDDM_LFBatwarnCFS_flg] -> DTC_Info/3
  DTC_Info/1 -> VDDM_LFBatwarnDTC_raw32/1  "VDDM_LFBatwarnDTC_raw32"
  Test Detection Criteria/1 -> [VDDM_LFBatwarnDet_flg]  "VDDM_LFBatwarnDet_flg"
  [VDDM_LFBatwarnDet_flg] -> DTC_Info/1
  [VDDM_LFBatwarnPass_flg] -> DTC_Info/2
  [DTC_clear_request] -> DTC_Info/4
  [VPMM_PowerSta_enum] -> Equal1/1
  Constant4/1 -> Switch3/3
  Constant5/1 -> Equal1/2
  Constant7/1 -> Equal5/2
  Logical Operator1/1 -> Switch3/2
  Equal5/1 -> Logical Operator1/1
  Equal1/1 -> Logical Operator1/2
  [VPMM_PowerSta_enum] -> Equal5/1
  Constant6/1 -> Test Detection Criteria/4
  Constant/1 -> Test Detection Criteria/3
  [task_time_s] -> Test Detection Criteria/2
  [VTPM_LFBatwarn_flg] -> Switch3/1
  [VPMM_PowerSta_enum] -> Equal3/1
  Equal2/1 -> Logical Operator4/2
  Constant8/1 -> Switch4/3
  Constant2/1 -> Equal2/2
  Constant3/1 -> Equal3/2
  [VPMM_PowerSta_enum] -> Equal2/1
  Equal3/1 -> Logical Operator4/1
  Logical Operator4/1 -> Switch4/2
  [VTPM_LFBatwarn_flg] -> Switch4/1
  VTPM_LFBatwarn_flg/1 -> [VTPM_LFBatwarn_flg]
  Switch3/1 -> [VDDM_LFBatwarnChk_flg], Switch6/3
  [DTC_clear_request] -> Switch6/2
  Constant12/1 -> Switch6/1
  Switch6/1 -> Test Detection Criteria/1
  Switch4/1 -> Timer1/2, Logical Operator6/1
  Equal6/1 -> SR_Latch1/1(set)
  Constant9/1 -> Equal6/2
  SR_Latch1/1(latched) -> [VDDM_LFBatwarnPass_flg]
  [VDDM_LFBatwarnChk_flg] -> SR_Latch1/2(reset)
  [task_time_s] -> Timer1/3
  Timer1/1 -> Equal6/1
  Constant15/1 -> Timer1/4
  Logical Operator6/1 -> Timer1/1
  Logical Operator2/1 -> Logical Operator19/3
  [DTC_clear_request] -> Logical Operator3/1, Logical Operator2/1
  Logical Operator5/1 -> SR_Latch4/2
  Constant1/1 -> DTC_Couter/3
  [DTC_clear_request] -> Logical Operator5/2
  [DTC_clear_request] -> Logical Operator7/2
  Logical Operator7/1 -> SR_Latch3/2

== system ddm/DDM/DDM/TPM/LFPressureLow ==
  note: Diagnostics and Fault Handling
  note: Release Condition After Decision
  note: Test Pass Criteria
  note: Test Detection Criteria
  task_time_s : Inport
  VPMM_PowerSta_enum : Inport  Port=2
  DTC_clear_request : Inport  Port=3
  VTPM_LFPressIndi_enum : Inport  Port=4
  Constant : Constant  Value=KDDM_LFPressIndiDTC_cnt
  Constant1 : Constant  Value=KDDM_LFPressIndiDTC_cnt
  Constant10 : Constant  Value=ENUM_POWERSTA_OFF
  Constant11 : Constant  Value=KDDM_LFPressIndiPassSW_flg
  Constant12 : Constant  Value=FALSE
  Constant13 : Constant  Value=KDDM_LFPressIndiCFSSW_flg
  Constant14 : Constant  Value=KDDM_LFPressIndiDFSSW_flg
  Constant15 : Constant  Value=KDDM_LFPressIndiPassTO_s
  Constant16 : Constant  Value=ENUM_PRESSINDI_LOW
  Constant17 : Constant  Value=ENUM_PRESSINDI_LOW
  Constant2 : Constant  Value=ENUM_POWERSTA_READY
  Constant24 : Constant  Value=TRUE
  Constant25 : Constant  Value=FALSE
  Constant3 : Constant  Value=ENUM_POWERSTA_ON
  Constant4 : Constant  Value=FALSE
  Constant46 : Constant  Value=KDDM_LFPressIndiDetSW_flg
  Constant5 : Constant  Value=ENUM_POWERSTA_READY
  Constant6 : Constant  Value=KDDM_LFPressIndiDetTO_s
  Constant7 : Constant  Value=ENUM_POWERSTA_ON
  Constant8 : Constant  Value=TRUE
  Constant9 : Constant  Value=KDDM_LFPressIndiPassTO_s
  DTC_Couter : hcu_lib/Basic_Blocks/DTC_Couter
  DTC_Info : hcu_lib/Basic_Blocks/DTC_Info
  Data Type Conversion1 : DataTypeConversion  OutDataTypeStr=uint8
  Equal{1..5,7..8} (7 alike) : RelationalOperator  Operator===  OutDataTypeStr=boolean  RndMeth=Simplest
  Equal6 : RelationalOperator  OutDataTypeStr=boolean  RndMeth=Simplest
  Logical Operator{1..2,4,7..8} (5 alike) : Logic  Operator=OR  AllPortsSameDT=off  OutDataTypeStr=boolean
  Logical Operator12 : Logic  AllPortsSameDT=off  OutDataTypeStr=boolean
  Logical Operator15 : Logic  AllPortsSameDT=off  OutDataTypeStr=boolean
  Logical Operator18 : Logic  AllPortsSameDT=off  OutDataTypeStr=boolean
  Logical Operator19 : Logic  Inputs=3  AllPortsSameDT=off  OutDataTypeStr=boolean
  Logical Operator3 : Logic  Operator=OR  Inputs=3  AllPortsSameDT=off  OutDataTypeStr=boolean
  Logical Operator5 : Logic  Operator=NOT  AllPortsSameDT=off  OutDataTypeStr=boolean
  Logical Operator6 : Logic  Operator=NOT  AllPortsSameDT=off  OutDataTypeStr=boolean
  Relay : Relay  OnSwitchValue=ONE_INT  OffSwitchValue=ZERO_INT
  SR_Latch1 : Subsystem  mask(SR_Latch){}
      mask help: SR latch function.
  SR_Latch3 : hcu_lib/Basic_Blocks/SR_Latch
  SR_Latch4 : hcu_lib/Basic_Blocks/SR_Latch
  Switch{2..4,6} (4 alike) : Switch  Criteria=u2 ~= 0
  Test Detection Criteria : hcu_lib/Basic_Blocks/Test Detection Criteria
  Timer1 : hcu_lib/Basic_Blocks/Timer
  VDDM_LFPressIndiDTC_raw32 : Outport
  wires:
  Logical Operator6/1 -> Timer1/1
  Constant15/1 -> Timer1/4
  Timer1/1 -> Equal6/1
  [task_time_s] -> Timer1/3
  [VDDM_LFPressIndiChk_flg] -> SR_Latch1/2(reset)
  SR_Latch1/1(latched) -> [VDDM_LFPressIndiPass_flg]
  Constant9/1 -> Equal6/2
  Equal6/1 -> SR_Latch1/1(set)
  Switch4/1 -> Logical Operator6/1, Timer1/2
  Switch6/1 -> Test Detection Criteria/1
  Constant12/1 -> Switch6/1
  [DTC_clear_request] -> Switch6/2
  Switch3/1 -> Switch6/3, [VDDM_LFPressIndiChk_flg]
  VTPM_LFPressIndi_enum/1 -> [VTPM_LFPressIndi_enum]
  Logical Operator4/1 -> Switch4/2
  Equal3/1 -> Logical Operator4/1
  [VPMM_PowerSta_enum] -> Equal2/1
  Constant3/1 -> Equal3/2
  Constant2/1 -> Equal2/2
  Constant8/1 -> Switch4/3
  Equal2/1 -> Logical Operator4/2
  [VPMM_PowerSta_enum] -> Equal3/1
  [task_time_s] -> Test Detection Criteria/2
  Constant/1 -> Test Detection Criteria/3
  Constant6/1 -> Test Detection Criteria/4
  [VPMM_PowerSta_enum] -> Equal5/1
  Equal1/1 -> Logical Operator1/2
  Equal5/1 -> Logical Operator1/1
  Logical Operator1/1 -> Switch3/2
  Constant7/1 -> Equal5/2
  Constant5/1 -> Equal1/2
  Constant4/1 -> Switch3/3
  [VPMM_PowerSta_enum] -> Equal1/1
  [DTC_clear_request] -> DTC_Info/4
  [VDDM_LFPressIndiPass_flg] -> DTC_Info/2
  [VDDM_LFPressIndiDet_flg] -> DTC_Info/1
  Test Detection Criteria/1 -> [VDDM_LFPressIndiDet_flg]  "VDDM_LFPressIndiDet_flg"
  DTC_Info/1 -> VDDM_LFPressIndiDTC_raw32/1  "VDDM_LFPressIndiDTC_raw32"
  [VDDM_LFPressIndiCFS_flg] -> DTC_Info/3
  [VPMM_PowerSta_enum] -> Equal4/1
  DTC_clear_request/1 -> [DTC_clear_request]
  [VDDM_LFPressIndiCFSRls_flg] -> Logical Operator3/3
  Logical Operator18/1 -> [VDDM_LFPressIndiCFS_flg]
  Constant14/1 -> Logical Operator12/1
  SR_Latch3/1 -> Logical Operator12/2
  Constant13/1 -> Logical Operator18/2
  Logical Operator12/1 -> [VDDM_LFPressIndiDFS_flg]
  SR_Latch4/1 -> Logical Operator18/1
  [VDDM_LFPressIndiCFSRls_flg] -> Logical Operator2/1
  [VDDM_LFPressIndiPass_flg] -> Logical Operator3/2
  DTC_Couter/1 -> SR_Latch4/1
  Data Type Conversion1/1 -> [VDDM_LFPressIndiDTC_cnt]  "VDDM_LFPressIndiDTC_cnt"
  Constant46/1 -> Logical Operator19/2
  Logical Operator19/1 -> DTC_Couter/1
  Constant11/1 -> Logical Operator15/2
  Logical Operator15/1 -> DTC_Couter/2
  Constant1/1 -> DTC_Couter/3
  DTC_Couter/2 -> Data Type Conversion1/1
  Relay/1 -> SR_Latch3/1
  [VDDM_LFPressIndiDet_flg] -> Logical Operator19/1
  Logical Operator3/1 -> Logical Operator15/1
  [VDDM_LFPressIndiCFS_flg] -> Logical Operator7/1
  [VDDM_LFPressIndiDTC_cnt] -> Relay/1
  Equal4/1 -> Logical Operator8/1
  Constant10/1 -> Equal4/2
  Constant24/1 -> Switch2/1
  [DTC_clear_request] -> Logical Operator8/2
  Switch2/1 -> [VDDM_LFPressIndiCFSRls_flg]
  Constant25/1 -> Switch2/3
  Logical Operator8/1 -> Switch2/2
  VPMM_PowerSta_enum/1 -> [VPMM_PowerSta_enum]
  task_time_s/1 -> [task_time_s]
  [VTPM_LFPressIndi_enum] -> Equal7/1
  Equal7/1 -> Switch3/1
  Constant16/1 -> Equal7/2
  Equal8/1 -> Switch4/1
  Constant17/1 -> Equal8/2
  [VTPM_LFPressIndi_enum] -> Equal8/1
  Logical Operator5/1 -> Logical Operator19/3
  [DTC_clear_request] -> Logical Operator3/1, Logical Operator5/1
  Logical Operator2/1 -> SR_Latch4/2
  [DTC_clear_request] -> Logical Operator2/2
  Logical Operator7/1 -> SR_Latch3/2
  [DTC_clear_request] -> Logical Operator7/2

== system ddm/DDM/DDM/TPM/LFSensorfail ==
  note: Diagnostics and Fault Handling
  note: Release Condition After Decision
  note: Test Pass Criteria
  note: Test Detection Criteria
  task_time_s : Inport
  VPMM_PowerSta_enum : Inport  Port=2
  DTC_clear_request : Inport  Port=3
  VTPM_LFSensorFail_flg : Inport  Port=4
  Constant : Constant  Value=KDDM_LFSensorFailDTC_cnt
  Constant1 : Constant  Value=KDDM_LFSensorFailDTC_cnt
  Constant10 : Constant  Value=ENUM_POWERSTA_OFF
  Constant11 : Constant  Value=KDDM_LFSensorFailPassSW_flg
  Constant12 : Constant  Value=FALSE
  Constant13 : Constant  Value=KDDM_LFSensorFailCFSSW_flg
  Constant14 : Constant  Value=KDDM_LFSensorFailDFSSW_flg
  Constant15 : Constant  Value=KDDM_LFSensorFailPassTO_s
  Constant2 : Constant  Value=ENUM_POWERSTA_READY
  Constant24 : Constant  Value=TRUE
  Constant25 : Constant  Value=FALSE
  Constant3 : Constant  Value=ENUM_POWERSTA_ON
  Constant4 : Constant  Value=FALSE
  Constant46 : Constant  Value=KDDM_LFSensorFailDetSW_flg
  Constant5 : Constant  Value=ENUM_POWERSTA_READY
  Constant6 : Constant  Value=KDDM_LFSensorFailDetTO_s
  Constant7 : Constant  Value=ENUM_POWERSTA_ON
  Constant8 : Constant  Value=TRUE
  Constant9 : Constant  Value=KDDM_LFSensorFailPassTO_s
  DTC_Couter : hcu_lib/Basic_Blocks/DTC_Couter
  DTC_Info : hcu_lib/Basic_Blocks/DTC_Info
  Data Type Conversion1 : DataTypeConversion  OutDataTypeStr=uint8
  Equal{1..5} (5 alike) : RelationalOperator  Operator===  OutDataTypeStr=boolean  RndMeth=Simplest
  Equal6 : RelationalOperator  OutDataTypeStr=boolean  RndMeth=Simplest
  Logical Operator{1,4..5,7..8} (5 alike) : Logic  Operator=OR  AllPortsSameDT=off  OutDataTypeStr=boolean
  Logical Operator12 : Logic  AllPortsSameDT=off  OutDataTypeStr=boolean
  Logical Operator15 : Logic  AllPortsSameDT=off  OutDataTypeStr=boolean
  Logical Operator18 : Logic  AllPortsSameDT=off  OutDataTypeStr=boolean
  Logical Operator19 : Logic  Inputs=3  AllPortsSameDT=off  OutDataTypeStr=boolean
  Logical Operator2 : Logic  Operator=NOT  AllPortsSameDT=off  OutDataTypeStr=boolean
  Logical Operator3 : Logic  Operator=OR  Inputs=3  AllPortsSameDT=off  OutDataTypeStr=boolean
  Logical Operator6 : Logic  Operator=NOT  AllPortsSameDT=off  OutDataTypeStr=boolean
  Relay : Relay  OnSwitchValue=ONE_INT  OffSwitchValue=ZERO_INT
  SR_Latch1 : Subsystem  mask(SR_Latch){}
      mask help: SR latch function.
  SR_Latch3 : hcu_lib/Basic_Blocks/SR_Latch
  SR_Latch4 : hcu_lib/Basic_Blocks/SR_Latch
  Switch{2..4,6} (4 alike) : Switch  Criteria=u2 ~= 0
  Test Detection Criteria : hcu_lib/Basic_Blocks/Test Detection Criteria
  Timer1 : hcu_lib/Basic_Blocks/Timer
  VDDM_LFSensorFailDTC_raw32 : Outport
  wires:
  Logical Operator6/1 -> Timer1/1
  Constant15/1 -> Timer1/4
  Timer1/1 -> Equal6/1
  [task_time_s] -> Timer1/3
  [VDDM_LFSensorFailChk_flg] -> SR_Latch1/2(reset)
  SR_Latch1/1(latched) -> [VDDM_LFSensorFailPass_flg]
  Constant9/1 -> Equal6/2
  Equal6/1 -> SR_Latch1/1(set)
  Switch4/1 -> Logical Operator6/1, Timer1/2
  Switch6/1 -> Test Detection Criteria/1
  Constant12/1 -> Switch6/1
  [DTC_clear_request] -> Switch6/2
  Switch3/1 -> Switch6/3, [VDDM_LFSensorFailChk_flg]
  VTPM_LFSensorFail_flg/1 -> [VTPM_LFSensorFail_flg]
  Logical Operator4/1 -> Switch4/2
  Equal3/1 -> Logical Operator4/1
  [VPMM_PowerSta_enum] -> Equal2/1
  Constant3/1 -> Equal3/2
  Constant2/1 -> Equal2/2
  Constant8/1 -> Switch4/3
  Equal2/1 -> Logical Operator4/2
  [VPMM_PowerSta_enum] -> Equal3/1
  [task_time_s] -> Test Detection Criteria/2
  Constant/1 -> Test Detection Criteria/3
  Constant6/1 -> Test Detection Criteria/4
  [VPMM_PowerSta_enum] -> Equal5/1
  Equal1/1 -> Logical Operator1/2
  Equal5/1 -> Logical Operator1/1
  Logical Operator1/1 -> Switch3/2
  Constant7/1 -> Equal5/2
  Constant5/1 -> Equal1/2
  Constant4/1 -> Switch3/3
  [VPMM_PowerSta_enum] -> Equal1/1
  [DTC_clear_request] -> DTC_Info/4
  [VDDM_LFSensorFailPass_flg] -> DTC_Info/2
  [VDDM_LFSensorFailDet_flg] -> DTC_Info/1
  Test Detection Criteria/1 -> [VDDM_LFSensorFailDet_flg]  "VDDM_LFSensorFailDet_flg"
  DTC_Info/1 -> VDDM_LFSensorFailDTC_raw32/1  "VDDM_LFSensorFailDTC_raw32"
  [VDDM_LFSensorFailCFS_flg] -> DTC_Info/3
  [VPMM_PowerSta_enum] -> Equal4/1
  DTC_clear_request/1 -> [DTC_clear_request]
  [VDDM_LFSensorFailCFSRls_flg] -> Logical Operator3/3
  Logical Operator18/1 -> [VDDM_LFSensorFailCFS_flg]
  Constant14/1 -> Logical Operator12/1
  SR_Latch3/1 -> Logical Operator12/2
  Constant13/1 -> Logical Operator18/2
  Logical Operator12/1 -> [VDDM_LFSensorFailDFS_flg]
  SR_Latch4/1 -> Logical Operator18/1
  [VDDM_LFSensorFailCFSRls_flg] -> Logical Operator5/1
  [VDDM_LFSensorFailPass_flg] -> Logical Operator3/2
  DTC_Couter/1 -> SR_Latch4/1
  Data Type Conversion1/1 -> [VDDM_LFSensorFailDTC_cnt]  "VDDM_LFSensorFailDTC_cnt"
  Constant46/1 -> Logical Operator19/2
  Logical Operator19/1 -> DTC_Couter/1
  Constant11/1 -> Logical Operator15/2
  Logical Operator15/1 -> DTC_Couter/2
  Constant1/1 -> DTC_Couter/3
  DTC_Couter/2 -> Data Type Conversion1/1
  Relay/1 -> SR_Latch3/1
  [VDDM_LFSensorFailDet_flg] -> Logical Operator19/1
  Logical Operator3/1 -> Logical Operator15/1
  [VDDM_LFSensorFailCFS_flg] -> Logical Operator7/1
  [VDDM_LFSensorFailDTC_cnt] -> Relay/1
  Equal4/1 -> Logical Operator8/1
  Constant10/1 -> Equal4/2
  Constant24/1 -> Switch2/1
  [DTC_clear_request] -> Logical Operator8/2
  Switch2/1 -> [VDDM_LFSensorFailCFSRls_flg]
  Constant25/1 -> Switch2/3
  Logical Operator8/1 -> Switch2/2
  VPMM_PowerSta_enum/1 -> [VPMM_PowerSta_enum]
  task_time_s/1 -> [task_time_s]
  [VTPM_LFSensorFail_flg] -> Switch3/1
  [VTPM_LFSensorFail_flg] -> Switch4/1
  Logical Operator2/1 -> Logical Operator19/3
  [DTC_clear_request] -> Logical Operator3/1, Logical Operator2/1
  Logical Operator5/1 -> SR_Latch4/2
  [DTC_clear_request] -> Logical Operator5/2
  Logical Operator7/1 -> SR_Latch3/2
  [DTC_clear_request] -> Logical Operator7/2
